simulink model "HSat_orbit"  (R2023a)
settings: Solver=FixedStepAuto  StartTime=0  StopTime=86400*900  MaxStep=3600  RelTol=1e-3  EnableMultiTasking=on
values from neighbouring files (symbols this model uses):
  ext_ENV_G = 6.674e-11    [HSat_op_setup.m]    (also in HSat_op_setup_merged_maria.m)
  ext_ENV_muEarth = 3.986005e14    (= 398600500000000)    [GEO_insertion_setup.m]    (also in HSat_op_setup.m; HSat_op_setup_merged_maria.m; init_orbit_analysis_with_drag_loss.m)
  ext_ENV_Re = 6.37813700*10^6    (= 6378137)    [HSat_op_setup.m]    (also in HSat_op_setup_merged_maria.m)
  ext_EOR_atmosphere_end = 1000e3    (= 1000000)    [HSat_op_setup.m]    (also in HSat_op_setup_merged_maria.m)
  ext_EOR_perigeeraise_end = 600e3    (= 600000)    [HSat_op_setup.m]    (also in HSat_op_setup_merged_maria.m)
  ext_Main_initDate_IC_T = sim_start    [HSat_op_setup.m]    (also in HSat_op_setup_merged_maria.m)
  ext_SC_activecorr_COE_ECI = [1, 1, 1, 0, 0, 0, 0, 0 ]    [HSat_op_setup.m]    (also in HSat_op_setup_merged_maria.m)
  ext_SC_balanced_COE_ECI = [ .500    0.70    1.100 1 1]    [HSat_op_setup.m]    (also in HSat_op_setup_merged_maria.m = [ 0.10 2.10 1.40    1.0000    1.0000]; launch_settings.m)
  ext_SC_cutofferror_COE_ECI = [150e3, .01, 0.1*pi/180, .1*pi/180,.1*pi/180, 0, 0, 0]    [HSat_op_setup.m]    (also in HSat_op_setup_merged_maria.m)
  ext_SC_init_COE_ECI = [a0,ecc0,i0,an0,ap0,tran0,eccan0,ma0]    [HSat_op_setup.m]    (also in HSat_op_setup_merged_maria.m)
  ext_SC_target_COE_ECI = [a1,ecc1,i1,an1,ap1,tran1,eccan1,ma1]    [HSat_op_setup.m]    (also in HSat_op_setup_merged_maria.m)
  ext_SC_target_lambda = 67*pi/180    (= 1.16937059884)    [HSat_op_setup.m]    (also in HSat_op_setup_merged_maria.m)
  sim_SC_init_CoG_EOR_dry = [-0.00448 0.00106 0.46931]    [HSat_op_setup.m]    (also in HSat_op_setup_merged_maria.m)
  sim_SC_init_CoG_propellant = [0 0 0.24758]    [HSat_op_setup.m]    (also in HSat_op_setup_merged_maria.m)
  sim_SC_init_dry_mass = sim_SC_init_wet_mass-sim_SC_init_propellant_mass    (= 727)    [HSat_op_setup.m]    (also in HSat_op_setup_merged_maria.m = 813.7)
  sim_SC_init_wet_mass = 750    [HSat_op_setup.m]    (also in HSat_op_setup_merged_maria.m)
  sim_thrust_force = [ ... (first row only)    [HSat_op_setup.m]    (also in HSat_op_setup_merged_maria.m)
  sim_thrust_massflow = [ ... (first row only)    [HSat_op_setup.m]    (also in HSat_op_setup_merged_maria.m)
  sim_thrust_vector = [ ... (first row only)    [HSat_op_setup.m]    (also in HSat_op_setup_merged_maria.m)
  sim_thruster_position = [ ... (first row only)    [HSat_op_setup.m]    (also in HSat_op_setup_merged_maria.m)
  sim_ts_save = 60    [HSat_op_setup.m]    (also in HSat_op_setup_merged_maria.m)
  third_body_jupiter = 1    [HSat_op_setup.m]    (also in HSat_op_setup_merged_maria.m)
  third_body_moon = 1    [HSat_op_setup.m]    (also in HSat_op_setup_merged_maria.m)
  third_body_sun = 1    [HSat_op_setup.m]    (also in HSat_op_setup_merged_maria.m)
libraries: aerolibutil x26, simulink x12, sharedtransform x7, sharedutil x4, Toolbox x3, matrix_library x1, simulink_extras x1
(part 2 of 5)

== system HSat_orbit/Subsystem1/Guidance/Subsystem1/Subsystem ==
  coe : Inport
  activecorr : Inport  Port=2
  coe1 : Inport  Port=3
  symelems : Inport  Port=4
  lambda1 : Inport  Port=5
  Abs : Abs  SaturateOnIntegerOverflow=off
  Bus Selector1 : BusSelector  OutputSignals=lambdadot,lambdaM
  Bus Selector2 : BusSelector  OutputSignals=sms
  Compare To Constant : simulink/Logic and Bit Operations/Compare To Constant  relop=<=  const=4  OutDataTypeStr=boolean
  Gain : Gain  Gain=180/pi
  Gain1 : Gain  Gain=180/pi
  Gain2 : Gain  Gain=180/pi
  Gain3 : Gain  Gain=.5
  Mux : Mux  Inputs=2
  Scope1 : Scope  NumInputPorts=3
  Scope2 : Scope  NumInputPorts=2
  Selector : Selector  InputPortWidth=8  IndexOptions=Index vector (dialog)  Indices=[2 3 4 5 6 7 8]  OutputSizes=1
  Subsystem1 : Subsystem
  Sum : Sum  Inputs=-+|
  plusminuspi : Subsystem
  NEARGEO : Outport
  ACTIVECORR : Outport  Port=2
  COE1 : Outport  Port=3
  wires:
  coe1/1 -> Selector/1
  coe/1 -> Bus Selector2/1
  lambda1/1 -> Sum/2
  symelems/1 -> Bus Selector1/1
  Abs/1 -> Compare To Constant/1
  Gain3/1 -> Gain1/1, Subsystem1/1(lambdadot_guide)
  Sum/1 -> plusminuspi/1(lambda)
  Selector/1 -> Mux/2
  Gain1/1 -> Scope1/2
  Gain2/1 -> Scope1/1
  Bus Selector1/1 -> Gain/1  "<lambdadot>"
  Bus Selector1/2 -> Sum/1  "<lambdaM>"
  Subsystem1/1(a_guide) -> Scope2/1, Mux/1
  Bus Selector2/1 -> Scope2/2  "<sms>"
  plusminuspi/1(lambdadot_guide) -> Gain2/1, Gain3/1
  Mux/1 -> COE1/1
  Gain/1 -> Scope1/3, Abs/1
  Compare To Constant/1 -> NEARGEO/1
  activecorr/1 -> ACTIVECORR/1

== system HSat_orbit/Subsystem1/Guidance/Subsystem1/perigeerraise ==
  coe : Inport
  "activecorr_coe " : Inport  Port=2
  Coe1 : Inport  Port=3
  Bus Selector : BusSelector  OutputSignals=sms
  Compare To Constant : simulink/Logic and Bit Operations/Compare To Constant  relop=<=  const=ext_EOR_perigeeraise_end  OutDataTypeStr=boolean
  Gain4 : Gain  Gain=[1 0 0 0 0 0 0 0]
  Gain5 : Gain  Gain=1.1
  Mux1 : Mux  Inputs=2
  Selector2 : Selector  InputPortWidth=8  IndexOptions=Index vector (dialog)  Indices=[2 3 4 5 6 7 8]  OutputSizes=1
  Subsystem2 : Subsystem
  Terminator : Terminator
  PERIGEEISLOW : Outport
  ACTIVECORR : Outport  Port=2
  COE1 : Outport  Port=3
  wires:
  Coe1/1 -> Selector2/1
  Compare To Constant/1 -> PERIGEEISLOW/1
  Subsystem2/2(Apogee altitude) -> Terminator/1
  "activecorr_coe "/1 -> Gain4/1
  Selector2/1 -> Mux1/2
  Subsystem2/1(Perigee altitude) -> Compare To Constant/1
  coe/1 -> Bus Selector/1, Subsystem2/1(COE)
  Gain4/1 -> ACTIVECORR/1
  Mux1/1 -> COE1/1
  Bus Selector/1 -> Gain5/1  "<sms>"
  Gain5/1 -> Mux1/1

== system HSat_orbit/Subsystem1/Navigation/Subsystem/Subsystem ==
  posECI : Inport
  velECI : Inport  Port=2
  Bus Creator : BusCreator  Inputs=11
  Demux : Demux  Outputs=11
  MATLAB Function : MATLAB Function  TreatAsAtomicUnit=on
  coe : Outport
  wires:
  posECI/1 -> MATLAB Function/1(r)
  Demux/10 -> Bus Creator/10  "truelong"
  Demux/1 -> Bus Creator/1  "sms"
  Demux/3 -> Bus Creator/3  "incl"
  Demux/7 -> Bus Creator/7  "eccan"
  Demux/9 -> Bus Creator/9  "arglat"
  Demux/4 -> Bus Creator/4  "raan"
  Demux/2 -> Bus Creator/2  "ecc"
  Demux/11 -> Bus Creator/11  "longper"
  Demux/6 -> Bus Creator/6  "truean"
  MATLAB Function/1(coe) -> Demux/1
  Bus Creator/1 -> coe/1  "coe"
  velECI/1 -> MATLAB Function/2(v)
  Demux/5 -> Bus Creator/5  "argp"
  Demux/8 -> Bus Creator/8  "meanan"

== system HSat_orbit/Subsystem1/Navigation/Subsystem/Subsystem2 ==
  jd : Inport
  epoch_jd : Inport  Port=2
  pos_ECI : Inport  Port=3
  vel_ECI : Inport  Port=4
  Bus Creator : BusCreator  Inputs=12
  Bus Creator1 : BusCreator  Inputs=10
  Bus Selector : BusSelector  OutputSignals=jd,epoch_jd,Raan,argp,nu,a,M,e,h
  Subsystem1 : Subsystem
  Subsystem7 : Subsystem
  Terminator : Terminator
  SyncElems : Outport
  wires:
  pos_ECI/1 -> Subsystem7/1(r)  "r"
  vel_ECI/1 -> Subsystem7/2(v)  "v"
  Subsystem7/9(e) -> Bus Creator/9
  Subsystem7/2(eabs) -> Bus Creator/2
  Subsystem7/10(h) -> Bus Creator/10
  Subsystem7/3(i) -> Bus Creator/3
  Subsystem7/5(argp) -> Bus Creator/5
  Subsystem7/4(Raan) -> Bus Creator/4
  Subsystem7/1(a) -> Bus Creator/1
  Subsystem7/6(nu) -> Bus Creator/6
  jd/1 -> Bus Creator/11  "jd"
  Bus Creator/1 -> Bus Selector/1
  Bus Selector/4 -> Subsystem1/4(<argp>)  "<argp>"
  Bus Selector/1 -> Subsystem1/1(<jd>)  "<jd>"
  Bus Selector/5 -> Subsystem1/5(<nu>)  "<nu>"
  Bus Selector/3 -> Subsystem1/3(<Raan>)  "<Raan>"
  Subsystem7/8(M) -> Bus Creator/8
  Subsystem7/7(E) -> Bus Creator/7
  Subsystem7/11(nu igen) -> Terminator/1
  epoch_jd/1 -> Bus Creator/12  "epoch_jd"
  Bus Selector/2 -> Subsystem1/2(epoch_jd)  "<epoch_jd>"
  Bus Selector/7 -> Subsystem1/7(M)  "<M>"
  Bus Selector/6 -> Subsystem1/6(a)  "<a>"
  Bus Selector/8 -> Subsystem1/8(e)  "<e>"
  Bus Selector/9 -> Subsystem1/9(h)  "<h>"
  Subsystem1/1(jd) -> Bus Creator1/1  "jd"
  Subsystem1/2(epochJd) -> Bus Creator1/2  "epochjd"
  Subsystem1/3(lambda) -> Bus Creator1/3  "lambda"
  Subsystem1/4(lambdaM) -> Bus Creator1/4  "lambdaM"
  Subsystem1/5(lambda0) -> Bus Creator1/5  "lambda0"
  Subsystem1/6(lambda_dot) -> Bus Creator1/6  "lambdadot"
  Subsystem1/7(ex) -> Bus Creator1/7  "ex"
  Subsystem1/9(ix) -> Bus Creator1/9  "ix"
  Bus Creator1/1 -> SyncElems/1
  Subsystem1/8(ey) -> Bus Creator1/8  "ey"
  Subsystem1/10(iy) -> Bus Creator1/10  "iy"

== system HSat_orbit/Subsystem1/Navigation/Subsystem8/Simplified Shadow Fraction ==
  note: Compute angular radius rho of Earth as viewed from ISS
  note: If dot product of normalized satellite position vector and sun vectors is smaller than cos rho then Earth is not blocking sun.
  x_sun_icrf : Inport  SampleTime=0
  X_icrf : Inport  Port=2
  Acos : Trigonometry  Operator=asin
  Acos1 : Trigonometry  Operator=cos
  Constant : Constant  Value=eps
  Constant1 : Constant  Value=eps
  Divide : Product  Inputs=/*
  Divide1 : Product  Inputs=*/
  Divide2 : Product  Inputs=/*
  Dot Product1 : DotProduct  OutDataTypeStr=Inherit: Inherit via internal rule
  Dot Product2 : DotProduct  OutDataTypeStr=Inherit: Inherit via internal rule
  Dot Product3 : DotProduct  OutDataTypeStr=Inherit: Inherit via internal rule
  Earth Radius : Constant  Value=ext_ENV_Re  VectorParams1D=off  SampleTime=0
  Gain : Gain  Gain=-1
  In Sun View : RelationalOperator  Operator=>  OutDataTypeStr=boolean  ZeroCross=off  RndMeth=Simplest  InputSameDT=off
  Max : MinMax  Function=max  Inputs=2
  Max1 : MinMax  Function=max  Inputs=2
  Sqrt1 : Sqrt
  Sqrt2 : Sqrt
  inView : Outport  SampleTime=0
  wires:
  Gain/1 -> Dot Product1/2, Divide/2, Dot Product1/1
  X_icrf/1 -> Divide2/2, Dot Product2/2, Dot Product2/1
  Earth Radius/1 -> Divide1/1
  Dot Product2/1 -> Sqrt1/1
  x_sun_icrf/1 -> Gain/1
  Max/1 -> Divide1/2, Divide2/1
  Divide1/1 -> Acos/1
  Acos/1 -> Acos1/1  "rho"
  Divide/1 -> Dot Product3/2
  Acos1/1 -> In Sun View/1
  Divide2/1 -> Dot Product3/1
  Dot Product3/1 -> In Sun View/2
  Dot Product1/1 -> Sqrt2/1
  Constant/1 -> Max/2
  In Sun View/1 -> inView/1
  Sqrt1/1 -> Max/1
  Sqrt2/1 -> Max1/1
  Max1/1 -> Divide/1
  Constant1/1 -> Max1/2

== system HSat_orbit/Subsystem1/Navigation/q_slo/VecNormalize ==
  In1 : Inport
  Constant : Constant
  Demux : Demux  Outputs=[-1 1]
  Divide : Product  Inputs=*/  OutDataTypeStr=double
  Ground : Ground
  Math Function : Math  Operator=square  SignedPower=on
  Math Function1 : Math  Operator=sqrt  SignedPower=on
  Mux : Mux  Inputs=2
  Mux1 : Mux  Inputs=2
  Product : Product  RndMeth=Zero
  Sum of Elements : Sum  Inputs=+
  Switch : Switch  Criteria=u2 > Threshold  Threshold=eps  SaturateOnIntegerOverflow=off  InputSameDT=off
  Out1 : Outport  VectorParamsAs1DForOutWhenUnconnected=off
  wires:
  Math Function/1 -> Sum of Elements/1
  Demux/1 -> Divide/1
  Constant/1 -> Mux1/2
  Mux1/1 -> Switch/3
  Divide/1 -> Out1/1
  Switch/1 -> Demux/1
  Mux/1 -> Switch/1
  Demux/2 -> Divide/2
  Product/1 -> Mux1/1
  In1/1 -> Product/1, Math Function/1, Mux/1
  Ground/1 -> Product/2
  Sum of Elements/1 -> Math Function1/1
  Math Function1/1 -> Mux/2, Switch/2

== system HSat_orbit/Subsystem1/Navigation/q_slo/VecNormalize1 ==
  In1 : Inport
  Constant : Constant
  Demux : Demux  Outputs=[-1 1]
  Divide : Product  Inputs=*/  OutDataTypeStr=double
  Ground : Ground
  Math Function : Math  Operator=square  SignedPower=on
  Math Function1 : Math  Operator=sqrt  SignedPower=on
  Mux : Mux  Inputs=2
  Mux1 : Mux  Inputs=2
  Product : Product  RndMeth=Zero
  Sum of Elements : Sum  Inputs=+
  Switch : Switch  Criteria=u2 > Threshold  Threshold=eps  SaturateOnIntegerOverflow=off  InputSameDT=off
  Out1 : Outport  VectorParamsAs1DForOutWhenUnconnected=off
  wires:
  Math Function/1 -> Sum of Elements/1
  Demux/1 -> Divide/1
  Constant/1 -> Mux1/2
  Mux1/1 -> Switch/3
  Divide/1 -> Out1/1
  Switch/1 -> Demux/1
  Mux/1 -> Switch/1
  Demux/2 -> Divide/2
  Product/1 -> Mux1/1
  In1/1 -> Product/1, Math Function/1, Mux/1
  Ground/1 -> Product/2
  Sum of Elements/1 -> Math Function1/1
  Math Function1/1 -> Mux/2, Switch/2

== system HSat_orbit/Subsystem1/Navigation/q_slo/VecNormalize2 ==
  In1 : Inport
  Constant : Constant
  Demux : Demux  Outputs=[-1 1]
  Divide : Product  Inputs=*/  OutDataTypeStr=double
  Ground : Ground
  Math Function : Math  Operator=square  SignedPower=on
  Math Function1 : Math  Operator=sqrt  SignedPower=on
  Mux : Mux  Inputs=2
  Mux1 : Mux  Inputs=2
  Product : Product  RndMeth=Zero
  Sum of Elements : Sum  Inputs=+
  Switch : Switch  Criteria=u2 > Threshold  Threshold=eps  SaturateOnIntegerOverflow=off  InputSameDT=off
  Out1 : Outport  VectorParamsAs1DForOutWhenUnconnected=off
  wires:
  Math Function/1 -> Sum of Elements/1
  Demux/1 -> Divide/1
  Constant/1 -> Mux1/2
  Mux1/1 -> Switch/3
  Divide/1 -> Out1/1
  Switch/1 -> Demux/1
  Mux/1 -> Switch/1
  Demux/2 -> Divide/2
  Product/1 -> Mux1/1
  In1/1 -> Product/1, Math Function/1, Mux/1
  Ground/1 -> Product/2
  Sum of Elements/1 -> Math Function1/1
  Math Function1/1 -> Mux/2, Switch/2

== system HSat_orbit/Subsystem1/Navigation/q_slo/VecNormalize3 ==
  In1 : Inport
  Constant : Constant
  Demux : Demux  Outputs=[-1 1]
  Divide : Product  Inputs=*/  OutDataTypeStr=double
  Ground : Ground
  Math Function : Math  Operator=square  SignedPower=on
  Math Function1 : Math  Operator=sqrt  SignedPower=on
  Mux : Mux  Inputs=2
  Mux1 : Mux  Inputs=2
  Product : Product  RndMeth=Zero
  Sum of Elements : Sum  Inputs=+
  Switch : Switch  Criteria=u2 > Threshold  Threshold=eps  SaturateOnIntegerOverflow=off  InputSameDT=off
  Out1 : Outport  VectorParamsAs1DForOutWhenUnconnected=off
  wires:
  Math Function/1 -> Sum of Elements/1
  Demux/1 -> Divide/1
  Constant/1 -> Mux1/2
  Mux1/1 -> Switch/3
  Divide/1 -> Out1/1
  Switch/1 -> Demux/1
  Mux/1 -> Switch/1
  Demux/2 -> Divide/2
  Product/1 -> Mux1/1
  In1/1 -> Product/1, Math Function/1, Mux/1
  Ground/1 -> Product/2
  Sum of Elements/1 -> Math Function1/1
  Math Function1/1 -> Mux/2, Switch/2

== system HSat_orbit/Subsystem1/Navigation/q_slo/Z x R ==
  a(1) a(2) a(3) : Inport
  b(1) b(2) b(3) : Inport  Port=2
  Product : Product  InputSameDT=on  SaturateOnIntegerOverflow=on  OutDataTypeStr=Inherit: Same as first input
  Product1 : Product  InputSameDT=on  SaturateOnIntegerOverflow=on  OutDataTypeStr=Inherit: Same as first input
  Selector : Selector  InputPortWidth=3  IndexOptions=Index vector (dialog)  Indices=[2 3 1]  OutputSizes=1
  Selector1 : Selector  InputPortWidth=3  IndexOptions=Index vector (dialog)  Indices=[3 1 2]  OutputSizes=1
  Selector2 : Selector  InputPortWidth=3  IndexOptions=Index vector (dialog)  Indices=[2 3 1]  OutputSizes=1
  Selector3 : Selector  InputPortWidth=3  IndexOptions=Index vector (dialog)  Indices=[3 1 2]  OutputSizes=1
  Sum : Sum  Inputs=+|-  InputSameDT=on  SaturateOnIntegerOverflow=on  OutDataTypeStr=Inherit: Same as first input
  c(1) c(2) c(3) : Outport  InitialOutput=0
  wires:
  Selector3/1 -> Product1/1
  Selector2/1 -> Product1/2
  Product1/1 -> Sum/2
  Selector1/1 -> Product/2
  Product/1 -> Sum/1
  a(1) a(2) a(3)/1 -> Selector3/1, Selector/1
  Selector/1 -> Product/1
  b(1) b(2) b(3)/1 -> Selector2/1, Selector1/1
  Sum/1 -> c(1) c(2) c(3)/1

== system HSat_orbit/Subsystem1/Navigation/q_slo/Z x Y ==
  a(1) a(2) a(3) : Inport
  b(1) b(2) b(3) : Inport  Port=2
  Product : Product  InputSameDT=on  SaturateOnIntegerOverflow=on  OutDataTypeStr=Inherit: Same as first input
  Product1 : Product  InputSameDT=on  SaturateOnIntegerOverflow=on  OutDataTypeStr=Inherit: Same as first input
  Selector : Selector  InputPortWidth=3  IndexOptions=Index vector (dialog)  Indices=[2 3 1]  OutputSizes=1
  Selector1 : Selector  InputPortWidth=3  IndexOptions=Index vector (dialog)  Indices=[3 1 2]  OutputSizes=1
  Selector2 : Selector  InputPortWidth=3  IndexOptions=Index vector (dialog)  Indices=[2 3 1]  OutputSizes=1
  Selector3 : Selector  InputPortWidth=3  IndexOptions=Index vector (dialog)  Indices=[3 1 2]  OutputSizes=1
  Sum : Sum  Inputs=+|-  InputSameDT=on  SaturateOnIntegerOverflow=on  OutDataTypeStr=Inherit: Same as first input
  c(1) c(2) c(3) : Outport  InitialOutput=0
  wires:
  Selector3/1 -> Product1/1
  Selector2/1 -> Product1/2
  Product1/1 -> Sum/2
  Selector1/1 -> Product/2
  Product/1 -> Sum/1
  a(1) a(2) a(3)/1 -> Selector3/1, Selector/1
  Selector/1 -> Product/1
  b(1) b(2) b(3)/1 -> Selector2/1, Selector1/1
  Sum/1 -> c(1) c(2) c(3)/1

== system HSat_orbit/Subsystem1/Subsystem4/EORattitude/Subsystem ==
  AmomECI : Inport
  q_eci2scb : Inport  Port=2
  EORthrustSCB : Inport  Port=3
  EORtorqueSCB : Inport  Port=4
  thrust_slo : Inport  Port=5
  q_slo2eci : Inport  Port=6
  sunv_eci : Inport  Port=7
  Quaternion Rotation1 : aerolibutil/Quaternion Rotation
  Subsystem1 : Subsystem
  Subsystem3 : Subsystem
  qECI2scb : Outport
  DoAMOM : Outport  Port=2
  NoAMOM : Outport  Port=3
  wires:
  q_slo2eci/1 -> Subsystem1/4(q_slo2eci)
  EORthrustSCB/1 -> Subsystem1/2(EORthrustSCB)
  sunv_eci/1 -> Subsystem1/5(sunv_eci)
  EORtorqueSCB/1 -> Subsystem3/2(EORtorqueSCB)
  thrust_slo/1 -> Subsystem1/3(thrust_slo)
  AmomECI/1 -> Quaternion Rotation1/2
  Subsystem1/1(qECI2scb) -> qECI2scb/1
  Subsystem3/3(FlipPlusMinus) -> Subsystem1/1(Flipsign)
  Quaternion Rotation1/1 -> Subsystem3/1(AmomSCB)  "amomscb"
  q_eci2scb/1 -> Quaternion Rotation1/1
  Subsystem3/1(DoAMOM) -> DoAMOM/1
  Subsystem3/2(NoAMOM) -> NoAMOM/1

== system HSat_orbit/Subsystem1/Subsystem4/EORattitude/Subsystem2 ==
  PPU1active : Inport
  AllThrustsSCB : Inport  Port=2
  PPU2active : Inport  Port=3
  AllTorquesSCB1 : Inport  Port=4
  PPU1ORTHR : Inport  Port=5
  PPU2ORTHR : Inport  Port=6
  Logical Operator : Logic  AllPortsSameDT=off  OutDataTypeStr=boolean
  Logical Operator1 : Logic  AllPortsSameDT=off  OutDataTypeStr=boolean
  Logical Operator2 : Logic  Operator=OR  AllPortsSameDT=off  OutDataTypeStr=boolean
  PPU1 : Subsystem
  PPU3 : Subsystem
  Product{,1..3} (4 alike) : Product
  Subsystem1 : Subsystem
  Sum1 : Sum  Inputs=++|
  Sum2 : Sum  Inputs=++|
  ActiveThrusters : Outport
  EORForceSCB : Outport  Port=2
  EORTorqueSCB : Outport  Port=3
  wires:
  AllTorquesSCB1/1 -> Subsystem1/2(AllTorquesSCB)
  Sum1/1 -> EORForceSCB/1
  Product2/1 -> Sum2/1
  PPU3/2(TorqueSCB) -> Product3/2
  PPU3/1(ForceSCB) -> Product1/2
  Sum2/1 -> EORTorqueSCB/1
  PPU1/1(ForceSCB) -> Product/2
  Subsystem1/2(TorquesORSCB) -> PPU3/3(TorqueORSCB), PPU1/3(TorqueORSCB)
  PPU1/2(TorqueSCB) -> Product2/2
  PPU2ORTHR/1 -> PPU3/2(OR ThrustNo)
  Logical Operator2/1 -> ActiveThrusters/1
  Subsystem1/1(ForceORSCB) -> PPU3/1(ForceORSCB), PPU1/1(ForceORSCB)
  PPU3/3(activethrusters) -> Logical Operator1/2
  AllThrustsSCB/1 -> Subsystem1/1(AllForcesSCB)
  Logical Operator/1 -> Logical Operator2/1
  PPU2active/1 -> Product3/1, Logical Operator1/1, Product1/1
  Product1/1 -> Sum1/2
  Logical Operator1/1 -> Logical Operator2/2
  Product/1 -> Sum1/1
  PPU1/3(activethrusters) -> Logical Operator/2
  PPU1active/1 -> Product2/1, Logical Operator/1, Product/1
  PPU1ORTHR/1 -> PPU1/2(OR ThrustNo)
  Product3/1 -> Sum2/2

== system HSat_orbit/Subsystem1/Subsystem4/EORattitude/Subsystem4 ==
  AmomECI : Inport
  EORthrustSCB : Inport  Port=2
  EORtorqueSCB : Inport  Port=3
  thrust_slo : Inport  Port=4
  q_slo2eci : Inport  Port=5
  sunv_eci : Inport  Port=6
  Delay1 : Delay  DelayLength=1  InitialConditionSource=Input port  InitialCondition=0
      settings: InputPortMap=u0,p4
  Quaternion Multiplication2 : aerolibutil/Quaternion Multiplication
  Quaternion Rotation1 : aerolibutil/Quaternion Rotation
  Subsystem1 : Subsystem
  Subsystem2 : Subsystem
  Subsystem3 : Subsystem
  Subsystem4 : Subsystem
  Switch1 : Switch  Criteria=u2 > Threshold  SaturateOnIntegerOverflow=off  InputSameDT=off
  qECI2scb : Outport
  DoAMOM : Outport  Port=2
  NoAMOM : Outport  Port=3
  wires:
  AmomECI/1 -> Quaternion Rotation1/2
  Quaternion Rotation1/1 -> Subsystem3/1(AmomSCB)  "amomscb"
  EORthrustSCB/1 -> Subsystem1/4(thrustscb), Subsystem2/1(thrustscb)  "thrustscb"
  EORtorqueSCB/1 -> Subsystem3/2(EORtorqueSCB)
  Subsystem3/1(Flipyaxis) -> Switch1/2
  Subsystem2/1(qflipscb) -> Switch1/1
  Subsystem4/1(qflipscb) -> Switch1/3
  Switch1/1 -> Quaternion Multiplication2/2
  Quaternion Multiplication2/1 -> Delay1/1, qECI2scb/1
  Delay1/1 -> Quaternion Rotation1/1
  Subsystem1/1(q*r) -> Delay1/2, Quaternion Multiplication2/1
  q_slo2eci/1 -> Subsystem1/1(q)
  thrust_slo/1 -> Subsystem1/2(vec)
  sunv_eci/1 -> Subsystem1/3(sunvECI)
  Subsystem3/2(DoAMOM) -> DoAMOM/1
  Subsystem3/3(NoAMOM) -> NoAMOM/1

== system HSat_orbit/Subsystem1/Subsystem4/Subsystem6/Subsystem2 ==
  PPU1active : Inport
  PPU2active : Inport  Port=2
  AllTorquesSCB : Inport  Port=3
  q_eci2scb_wanted : Inport  Port=4
  WantedTorqueECI : Inport  Port=5
  sunv : Inport  Port=6
  Multiport Switch : MultiPortSwitch  SaturateOnIntegerOverflow=off  InputSameDT=off
  Multiport Switch1 : MultiPortSwitch  SaturateOnIntegerOverflow=off  InputSameDT=off
  PPU1 : Subsystem
  PPU1+2 : Subsystem
  PPU2 : Subsystem
  Subsystem : Subsystem
  Subsystem1 : Subsystem
  Sum1 : Sum  Inputs=++|
  ActiveThrusters : Outport
  q_eci2scb : Outport  Port=2
  wires:
  Multiport Switch1/1 -> ActiveThrusters/1
  PPU1active/1 -> Sum1/1
  PPU2active/1 -> Sum1/2
  PPU1+2/2(activethrusters) -> Multiport Switch1/4
  PPU1/2(activethrusters) -> Multiport Switch1/2
  PPU1/1(torqueSCB) -> Multiport Switch/2  "torquescb"
  PPU1+2/1(torqueSCB) -> Multiport Switch/4  "torquescb"
  PPU2/2(activethrusters) -> Multiport Switch1/3
  Sum1/1 -> Multiport Switch/1, Multiport Switch1/1
  WantedTorqueECI/1 -> Subsystem1/2(WantedTorqueECI), PPU1+2/2(WantedTorqueECI), PPU2/2(WantedTorqueECI), PPU1/2(WantedTorqueECI)
  PPU2/1(torqueSCB) -> Multiport Switch/3  "torquescb"
  Subsystem/1(TorqueSKECI) -> PPU1+2/1(TorqueSKECI), PPU2/1(TorqueSKECI), PPU1/1(TorqueSKECI)
  q_eci2scb_wanted/1 -> Subsystem/2(q_eci2scb_wanted)
  AllTorquesSCB/1 -> Subsystem/1(AllTorquesSCB)
  Subsystem1/1(q_eci2scb) -> q_eci2scb/1
  sunv/1 -> Subsystem1/3(sunvECI)
  Multiport Switch/1 -> Subsystem1/1(TorqueSCB)

== system HSat_orbit/Subsystem1/Subsystem4/TorquesAndForces/Subsystem ==
  SC_mass : Inport
  Constant1 : Constant  Value=sim_SC_init_CoG_EOR_dry
  Constant2 : Constant  Value=sim_SC_init_CoG_propellant
  Constant3 : Constant  Value=sim_SC_init_wet_mass
  Constant4 : Constant  Value=sim_SC_init_dry_mass
  Divide : Product  Inputs=/*
  Product : Product
  Product1 : Product
  Reshape : Reshape  OutputDimensionality=Row vector (2-D)
  Sum : Sum  Inputs=+-|
  Sum1 : Sum  Inputs=+|+
  SC_CoG : Outport
  wires:
  Constant4/1 -> Sum/2
  Product1/1 -> Sum1/2
  Constant3/1 -> Product1/1
  SC_mass/1 -> Divide/1, Sum/1
  Constant1/1 -> Product1/2
  Product/1 -> Sum1/1
  Sum1/1 -> Divide/2
  Constant2/1 -> Product/2
  Sum/1 -> Product/1
  Divide/1 -> Reshape/1
  Reshape/1 -> SC_CoG/1

== system HSat_orbit/Subsystem1/Dynamics/Subsystem/3 body perturbation legendre polynomial/Subsystem1 ==
  sat : Inport
  3 body : Inport  Port=2
  mass : Inport  Port=3
  Legendre deg : Inport  Port=4
  Constant : Constant  Value=6.6743e-11
  Divide : Product  Inputs=/*
  Divide1 : Product  Inputs=*/
  Dot Product : DotProduct  OutDataTypeStr=Inherit: Inherit via internal rule
  Dot Product1 : DotProduct  OutDataTypeStr=Inherit: Inherit via internal rule
  Dot Product2 : DotProduct  OutDataTypeStr=Inherit: Inherit via internal rule
  MATLAB Function : MATLAB Function  TreatAsAtomicUnit=on
  Product{,1..3} (4 alike) : Product
  Sqrt : Sqrt
  Sqrt1 : Sqrt
  Subtract : Sum  Inputs=-+
  Subtract1 : Sum  Inputs=+-
  cos angle : Subsystem
  Out1 : Outport
  wires:
  sat/1 -> cos angle/1(sat), Subtract/2, Subtract1/2, Dot Product2/2, Dot Product2/1  "r_sat"
  3 body/1 -> Dot Product1/1, Dot Product/2, Dot Product/1, Dot Product1/2, Subtract1/1, cos angle/2(3 body)  "r_3body"
  cos angle/1(cos angle) -> MATLAB Function/1(costheta)
  Legendre deg/1 -> MATLAB Function/2(degree)
  Divide/1 -> MATLAB Function/3(h)
  mass/1 -> Product/2
  Constant/1 -> Product/1
  Product/1 -> Divide1/1  "mu_3body"
  Divide1/1 -> Product1/1
  Product1/1 -> Out1/1
  MATLAB Function/1(beta) -> Product2/1
  Subtract1/1 -> Product2/2  "r_sat3body"
  Product2/1 -> Subtract/1
  Subtract/1 -> Product1/2
  Dot Product/1 -> Product3/1
  Product3/1 -> Divide1/2
  Dot Product1/1 -> Sqrt/1
  Sqrt/1 -> Divide/1, Product3/2  "| r_3body |"
  Dot Product2/1 -> Sqrt1/1
  Sqrt1/1 -> Divide/2  "| r_sat |"

== system HSat_orbit/Subsystem1/Dynamics/Subsystem/3 body perturbation legendre polynomial/Subsystem2 ==
  sat : Inport
  3 body : Inport  Port=2
  mass : Inport  Port=3
  Legendre deg : Inport  Port=4
  Constant : Constant  Value=ext_ENV_G
  Divide : Product  Inputs=/*
  Divide1 : Product  Inputs=*/
  Dot Product : DotProduct  OutDataTypeStr=Inherit: Inherit via internal rule
  Dot Product1 : DotProduct  OutDataTypeStr=Inherit: Inherit via internal rule
  Dot Product2 : DotProduct  OutDataTypeStr=Inherit: Inherit via internal rule
  MATLAB Function : MATLAB Function  TreatAsAtomicUnit=on
  Product{,1..3} (4 alike) : Product
  Sqrt : Sqrt
  Sqrt1 : Sqrt
  Subtract : Sum  Inputs=-+
  Subtract1 : Sum  Inputs=+-
  cos angle : Subsystem
  Out1 : Outport
  wires:
  sat/1 -> cos angle/1(sat), Subtract/2, Subtract1/2, Dot Product2/2, Dot Product2/1  "r_sat"
  3 body/1 -> Dot Product1/1, Dot Product/2, Dot Product/1, Dot Product1/2, Subtract1/1, cos angle/2(3 body)  "r_3body"
  cos angle/1(cos angle) -> MATLAB Function/1(costheta)
  Legendre deg/1 -> MATLAB Function/2(degree)
  Divide/1 -> MATLAB Function/3(h)
  mass/1 -> Product/2
  Constant/1 -> Product/1
  Product/1 -> Divide1/1  "mu_3body"
  Divide1/1 -> Product1/1
  Product1/1 -> Out1/1
  MATLAB Function/1(beta) -> Product2/1
  Subtract1/1 -> Product2/2  "r_sat3body"
  Product2/1 -> Subtract/1
  Subtract/1 -> Product1/2
  Dot Product/1 -> Product3/1
  Product3/1 -> Divide1/2
  Dot Product1/1 -> Sqrt/1
  Sqrt/1 -> Divide/1, Product3/2  "| r_3body |"
  Dot Product2/1 -> Sqrt1/1
  Sqrt1/1 -> Divide/2  "| r_sat |"

== system HSat_orbit/Subsystem1/Dynamics/Subsystem/3 body perturbation legendre polynomial/Subsystem3 ==
  sat : Inport
  3 body : Inport  Port=2
  mass : Inport  Port=3
  Legendre deg : Inport  Port=4
  Constant : Constant  Value=6.6743e-11
  Divide : Product  Inputs=/*
  Divide1 : Product  Inputs=*/
  Dot Product : DotProduct  OutDataTypeStr=Inherit: Inherit via internal rule
  Dot Product1 : DotProduct  OutDataTypeStr=Inherit: Inherit via internal rule
  Dot Product2 : DotProduct  OutDataTypeStr=Inherit: Inherit via internal rule
  MATLAB Function : MATLAB Function  TreatAsAtomicUnit=on
  Product{,1..3} (4 alike) : Product
  Sqrt : Sqrt
  Sqrt1 : Sqrt
  Subtract : Sum  Inputs=-+
  Subtract1 : Sum  Inputs=+-
  cos angle : Subsystem
  Out1 : Outport
  wires:
  sat/1 -> cos angle/1(sat), Subtract/2, Subtract1/2, Dot Product2/2, Dot Product2/1  "r_sat"
  3 body/1 -> Dot Product1/1, Dot Product/2, Dot Product/1, Dot Product1/2, Subtract1/1, cos angle/2(3 body)  "r_3body"
  cos angle/1(cos angle) -> MATLAB Function/1(costheta)
  Legendre deg/1 -> MATLAB Function/2(degree)
  Divide/1 -> MATLAB Function/3(h)
  mass/1 -> Product/2
  Constant/1 -> Product/1
  Product/1 -> Divide1/1  "mu_3body"
  Divide1/1 -> Product1/1
  Product1/1 -> Out1/1
  MATLAB Function/1(beta) -> Product2/1
  Subtract1/1 -> Product2/2  "r_sat3body"
  Product2/1 -> Subtract/1
  Subtract/1 -> Product1/2
  Dot Product/1 -> Product3/1
  Product3/1 -> Divide1/2
  Dot Product1/1 -> Sqrt/1
  Sqrt/1 -> Divide/1, Product3/2  "| r_3body |"
  Dot Product2/1 -> Sqrt1/1
  Sqrt1/1 -> Divide/2  "| r_sat |"

== system HSat_orbit/Subsystem1/Guidance/Subsystem1/Subsystem/Subsystem1 ==
  lambdadot_guide : Inport
  Constant1 : Constant  Value=2*pi
  Constant5 : Constant  Value=2*pi*86164
  Constant6 : Constant  Value=ext_ENV_muEarth
  Constant7 : Constant  Value=1/3
  Constant8 : Constant  Value=2*pi
  Divide1 : Product  Inputs=**
  Divide2 : Product  Inputs=*/
  Divide3 : Product  Inputs=*/
  Gain : Gain
  Math Function4 : Math  Operator=square
  Math Function5 : Math  Operator=pow
  Subtract1 : Sum
  a_guide : Outport
  wires:
  Constant6/1 -> Divide1/2
  Divide1/1 -> Math Function5/1
  Constant7/1 -> Math Function5/2
  lambdadot_guide/1 -> Gain/1
  Math Function4/1 -> Divide1/1
  Math Function5/1 -> a_guide/1
  Constant8/1 -> Subtract1/2
  Subtract1/1 -> Divide2/2
  Divide2/1 -> Divide3/1  "T-period"
  Constant5/1 -> Divide2/1
  Constant1/1 -> Divide3/2
  Divide3/1 -> Math Function4/1  "T-period"
  Gain/1 -> Subtract1/1

== system HSat_orbit/Subsystem1/Guidance/Subsystem1/Subsystem/plusminuspi ==
  lambda : Inport
  Constant1 : Constant  Value=2*pi
  Constant2 : Constant  Value=2*pi
  Constant4 : Constant  Value=2*pi
  Constant5 : Constant  Value=pi
  Math Function1 : Math  Operator=mod
  Math Function2 : Math  Operator=mod
  Math Function3 : Math  Operator=mod
  Sum11 : Sum  Inputs=|+-
  Sum12 : Sum  Inputs=|++
  lambdadot_guide : Outport
  wires:
  Sum11/1 -> Math Function1/1
  Sum12/1 -> Math Function3/1
  Math Function3/1 -> Sum11/1
  Constant5/1 -> Sum12/2, Sum11/2
  Constant4/1 -> Math Function3/2
  lambda/1 -> Math Function2/1
  Constant1/1 -> Math Function1/2
  Math Function2/1 -> Sum12/1
  Constant2/1 -> Math Function2/2
  Math Function1/1 -> lambdadot_guide/1

== system HSat_orbit/Subsystem1/Guidance/Subsystem1/perigeerraise/Subsystem2 ==
  COE : Inport
  Bus Selector : BusSelector  OutputSignals=sms,ecc
  Constant : Constant
  Constant1 : Constant  Value=ext_ENV_Re
  Product : Product
  Product1 : Product
  Sum : Sum  Inputs=|-+
  Sum1 : Sum  Inputs=|++
  Sum2 : Sum  Inputs=|+-
  Sum3 : Sum  Inputs=|+-
  Perigee altitude : Outport
  Apogee altitude : Outport  Port=2
  wires:
  Product1/1 -> Sum3/1
  COE/1 -> Bus Selector/1
  Sum1/1 -> Product1/2
  Product/1 -> Sum2/1
  Constant/1 -> Sum1/2, Sum/2
  Sum/1 -> Product/2
  Bus Selector/1 -> Product1/1, Product/1  "<sms>"
  Sum2/1 -> Perigee altitude/1
  Sum3/1 -> Apogee altitude/1
  Constant1/1 -> Sum2/2, Sum3/2
  Bus Selector/2 -> Sum/1, Sum1/1  "<ecc>"

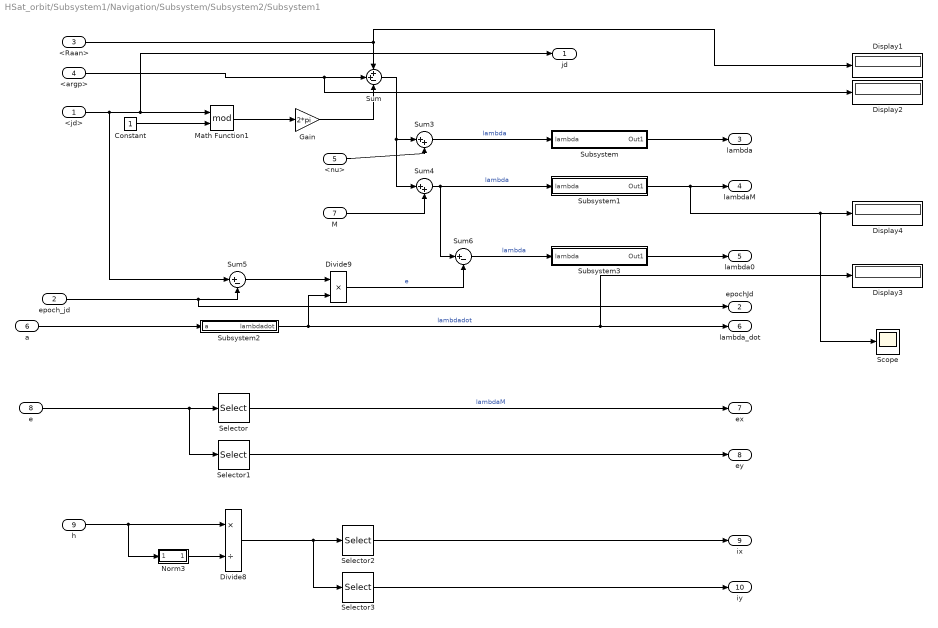
== system HSat_orbit/Subsystem1/Navigation/Subsystem/Subsystem2/Subsystem1 ==
  <jd> : Inport
  epoch_jd : Inport  Port=2
  <Raan> : Inport  Port=3
  <argp> : Inport  Port=4
  <nu> : Inport  Port=5
  a : Inport  Port=6
  M : Inport  Port=7
  e : Inport  Port=8
  h : Inport  Port=9
  Constant : Constant
  Display{1..4} (4 alike) : Display
  Divide8 : Product  Inputs=*/
  Divide9 : Product  Inputs=**
  Gain : Gain  Gain=2*pi
  Math Function1 : Math  Operator=mod
  Norm3 : Subsystem  Tag=||u||
      mask Display: disp('||u||')
  Scope : Scope
  Selector : Selector  InputPortWidth=3  IndexOptions=Index vector (dialog)  Indices=[1]  OutputSizes=1
  Selector1 : Selector  InputPortWidth=3  IndexOptions=Index vector (dialog)  Indices=[2]  OutputSizes=1
  Selector2 : Selector  InputPortWidth=3  IndexOptions=Index vector (dialog)  Indices=[1]  OutputSizes=1
  Selector3 : Selector  InputPortWidth=3  IndexOptions=Index vector (dialog)  Indices=[2]  OutputSizes=1
  Subsystem : Subsystem
  Subsystem1 : Subsystem
  Subsystem2 : Subsystem
  Subsystem3 : Subsystem
  Sum : Sum  Inputs=++-
  Sum3 : Sum  Inputs=|++
  Sum4 : Sum  Inputs=|++
  Sum5 : Sum  Inputs=|+-
  Sum6 : Sum  Inputs=|+-
  jd : Outport
  epochJd : Outport  Port=2
  lambda : Outport  Port=3
  lambdaM : Outport  Port=4
  lambda0 : Outport  Port=5
  lambda_dot : Outport  Port=6
  ex : Outport  Port=7
  ey : Outport  Port=8
  ix : Outport  Port=9
  iy : Outport  Port=10
  wires:
  <Raan>/1 -> Sum/1, Display1/1
  <nu>/1 -> Sum3/2
  Gain/1 -> Sum/3
  Math Function1/1 -> Gain/1
  <jd>/1 -> Sum5/1, Math Function1/1, jd/1
  Constant/1 -> Math Function1/2
  a/1 -> Subsystem2/1(a)
  Sum/1 -> Sum4/1, Sum3/1
  M/1 -> Sum4/2
  epoch_jd/1 -> epochJd/1, Sum5/2
  Sum5/1 -> Divide9/1
  Subsystem2/1(lambdadot) -> Divide9/2, Display3/1, lambda_dot/1  "lambdadot"
  Divide9/1 -> Sum6/2  "e"
  e/1 -> Selector1/1, Selector/1
  Selector1/1 -> ey/1
  Selector/1 -> ex/1  "lambdaM"
  Divide8/1 -> Selector3/1, Selector2/1
  Selector3/1 -> iy/1
  Selector2/1 -> ix/1
  Norm3/1(Out1) -> Divide8/2
  h/1 -> Norm3/1(In1), Divide8/1
  Sum4/1 -> Sum6/1, Subsystem1/1(lambda)  "lambda"
  Sum3/1 -> Subsystem/1(lambda)  "lambda"
  Subsystem/1(Out1) -> lambda/1
  Subsystem1/1(Out1) -> Scope/1, Display4/1, lambdaM/1
  Sum6/1 -> Subsystem3/1(lambda)  "lambda"
  Subsystem3/1(Out1) -> lambda0/1
  <argp>/1 -> Display2/1, Sum/2

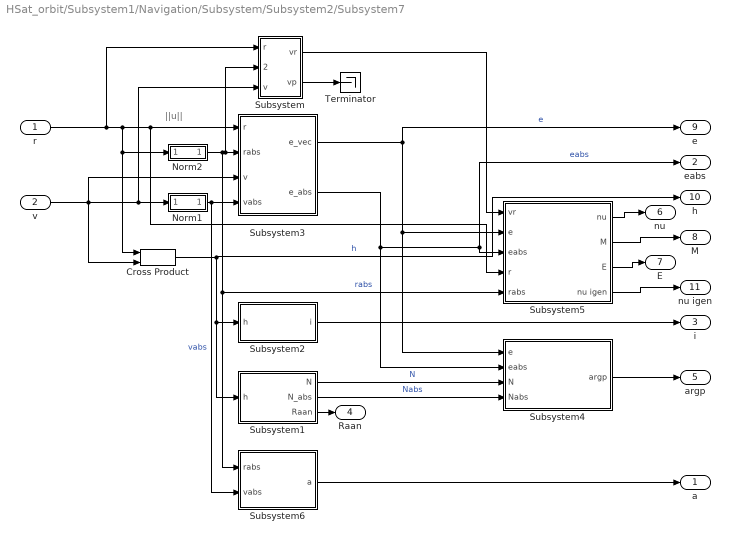
== system HSat_orbit/Subsystem1/Navigation/Subsystem/Subsystem2/Subsystem7 ==
  note: ||u||
  r : Inport
  v : Inport  Port=2
  Cross Product : matrix_library/Cross Product
  Norm1 : Subsystem  Tag=||u||
      mask Display: disp('||u||')
  Norm2 : Subsystem  Tag=||u||
      mask Display: disp('||u||')
  Subsystem : Subsystem
  Subsystem1 : Subsystem
  Subsystem2 : Subsystem
  Subsystem3 : Subsystem
  Subsystem4 : Subsystem
  Subsystem5 : Subsystem
  Subsystem6 : Subsystem
  Terminator : Terminator
  a : Outport
  eabs : Outport  Port=2
  i : Outport  Port=3
  Raan : Outport  Port=4
  argp : Outport  Port=5
  nu : Outport  Port=6
  E : Outport  Port=7
  M : Outport  Port=8
  e : Outport  Port=9
  h : Outport  Port=10
  nu igen : Outport  Port=11
  wires:
  Subsystem5/1(nu) -> nu/1
  Subsystem1/3(Raan) -> Raan/1
  Subsystem1/1(N) -> Subsystem4/3(N)  "N"
  Subsystem6/1(a) -> a/1
  Subsystem1/2(N_abs) -> Subsystem4/4(Nabs)  "Nabs"
  Subsystem3/1(e_vec) -> e/1, Subsystem4/1(e), Subsystem5/2(e)  "e"
  Subsystem4/1(argp) -> argp/1
  Norm1/1(Out1) -> Subsystem6/2(vabs), Subsystem3/4(vabs)  "vabs"
  Subsystem2/1(i) -> i/1
  Cross Product/1 -> Subsystem1/1(h), Subsystem2/1(h), h/1  "h"
  v/1 -> Cross Product/2, Subsystem3/3(v), Subsystem/3(v), Norm1/1(In1)
  Subsystem3/2(e_abs) -> eabs/1, Subsystem5/3(eabs), Subsystem4/2(eabs)  "eabs"
  Norm2/1(Out1) -> Subsystem/2(rabs), Subsystem3/2(rabs), Subsystem6/1(rabs), Subsystem5/5(rabs)  "rabs"
  Subsystem5/2(M) -> M/1
  Subsystem5/4(nu igen) -> nu igen/1
  Subsystem5/3(E) -> E/1
  r/1 -> Subsystem/1(r), Norm2/1(In1), Cross Product/1, Subsystem5/4(r), Subsystem3/1(r)
  Subsystem/1(vr) -> Subsystem5/1(vr)
  Subsystem/2(vp) -> Terminator/1

== system HSat_orbit/Subsystem1/Subsystem4/EORattitude/Subsystem/Subsystem1 ==
  note: the scbp fram is an intemediate frame where:
      | - z is aligned with the resutling thrust,
      | - y is the normalised cross product between the sun vector and z
      | - x completes the orthogonal system
  Flipsign : Inport
  EORthrustSCB : Inport  Port=2
  thrust_slo : Inport  Port=3
  q_slo2eci : Inport  Port=4
  sunv_eci : Inport  Port=5
  Quaternion Inverse : aerolibutil/Quaternion Inverse
  Quaternion Multiplication : aerolibutil/Quaternion Multiplication
  Quaternion Rotation : aerolibutil/Quaternion Rotation
  Subsystem : Subsystem
  q_scb_calc : Subsystem
  qECI2scb : Outport
  wires:
  thrust_slo/1 -> Quaternion Rotation/2
  q_slo2eci/1 -> Quaternion Inverse/1
  sunv_eci/1 -> q_scb_calc/2(sunvECI)
  Quaternion Rotation/1 -> q_scb_calc/1(EORthrustECI)  "vec_eci"
  Quaternion Inverse/1 -> Quaternion Rotation/1
  q_scb_calc/1(qECI2scbp) -> Quaternion Multiplication/1
  Flipsign/1 -> Subsystem/2(Flipsign)
  Subsystem/1(qscbp2scb) -> Quaternion Multiplication/2
  EORthrustSCB/1 -> Subsystem/1(EORthrustSCB)  "thrustscb"
  Quaternion Multiplication/1 -> qECI2scb/1

== system HSat_orbit/Subsystem1/Subsystem4/EORattitude/Subsystem/Subsystem3 ==
  AmomSCB : Inport
  EORtorqueSCB : Inport  Port=2
  FlipSatellite : Subsystem
  Subsystem : Subsystem
  DoAMOM : Outport
  NoAMOM : Outport  Port=2
  FlipPlusMinus : Outport  Port=3
  wires:
  AmomSCB/1 -> FlipSatellite/1(AmomSCB)
  Subsystem/1(FlipPlusMinus) -> FlipPlusMinus/1
  EORtorqueSCB/1 -> FlipSatellite/2(EORtorqueSCB)
  FlipSatellite/1(FlipSatellite_bool) -> Subsystem/1(FlipNow)
  FlipSatellite/2(DoAMOM) -> DoAMOM/1
  FlipSatellite/3(NoAMOM) -> NoAMOM/1

== system HSat_orbit/Subsystem1/Subsystem4/EORattitude/Subsystem2/PPU1 ==
  ForceORSCB : Inport
  OR ThrustNo : Inport  Port=2
  TorqueORSCB : Inport  Port=3
  Constant : Constant  Value=[0 0 0 0 0 0 0 0 1 0 0]
  Constant1 : Constant  Value=[0 0 0 0 0 0 0 0 0 0 0]
  Constant2 : Constant  Value=[0 0 0 0 0 0 0 0 0 0 1]
  Demux : Demux  Outputs=3
  Demux1 : Demux  Outputs=3
  Multiport Switch : MultiPortSwitch  SaturateOnIntegerOverflow=off  InputSameDT=off
  Multiport Switch1 : MultiPortSwitch  SaturateOnIntegerOverflow=off  InputSameDT=off
  Multiport Switch2 : MultiPortSwitch  SaturateOnIntegerOverflow=off  InputSameDT=off
  ForceSCB : Outport
  TorqueSCB : Outport  Port=2
  activethrusters : Outport  Port=3
  wires:
  ForceORSCB/1 -> Demux/1
  Demux/1 -> Multiport Switch/2
  Demux/2 -> Multiport Switch/3
  Demux/3 -> Multiport Switch/4
  Multiport Switch/1 -> ForceSCB/1
  Constant1/1 -> Multiport Switch1/3
  Multiport Switch1/1 -> activethrusters/1
  Constant/1 -> Multiport Switch1/2
  Constant2/1 -> Multiport Switch1/4
  Multiport Switch2/1 -> TorqueSCB/1
  TorqueORSCB/1 -> Demux1/1
  Demux1/3 -> Multiport Switch2/4
  Demux1/1 -> Multiport Switch2/2
  OR ThrustNo/1 -> Multiport Switch1/1, Multiport Switch2/1, Multiport Switch/1
  Demux1/2 -> Multiport Switch2/3

== system HSat_orbit/Subsystem1/Subsystem4/EORattitude/Subsystem2/PPU3 ==
  ForceORSCB : Inport
  OR ThrustNo : Inport  Port=2
  TorqueORSCB : Inport  Port=3
  Constant : Constant  Value=[0 0 0 0 0 0 0 0 0 0 0]
  Constant1 : Constant  Value=[0 0 0 0 0 0 0 0 0 1 0]
  Constant2 : Constant  Value=[0 0 0 0 0 0 0 0 0 0 1]
  Demux : Demux  Outputs=3
  Demux1 : Demux  Outputs=3
  Multiport Switch : MultiPortSwitch  SaturateOnIntegerOverflow=off  InputSameDT=off
  Multiport Switch1 : MultiPortSwitch  SaturateOnIntegerOverflow=off  InputSameDT=off
  Multiport Switch2 : MultiPortSwitch  SaturateOnIntegerOverflow=off  InputSameDT=off
  ForceSCB : Outport
  TorqueSCB : Outport  Port=2
  activethrusters : Outport  Port=3
  wires:
  ForceORSCB/1 -> Demux/1
  Demux/1 -> Multiport Switch/2
  Demux/2 -> Multiport Switch/3
  Demux/3 -> Multiport Switch/4
  Multiport Switch/1 -> ForceSCB/1
  Constant1/1 -> Multiport Switch1/3
  Multiport Switch1/1 -> activethrusters/1
  Constant/1 -> Multiport Switch1/2
  Constant2/1 -> Multiport Switch1/4
  Multiport Switch2/1 -> TorqueSCB/1
  TorqueORSCB/1 -> Demux1/1
  Demux1/3 -> Multiport Switch2/4
  Demux1/1 -> Multiport Switch2/2
  OR ThrustNo/1 -> Multiport Switch1/1, Multiport Switch2/1, Multiport Switch/1
  Demux1/2 -> Multiport Switch2/3

== system HSat_orbit/Subsystem1/Subsystem4/EORattitude/Subsystem2/Subsystem1 ==
  AllForcesSCB : Inport
  AllTorquesSCB : Inport  Port=2
  ForceSCBOR1 : Selector  NumberOfDimensions=2  InputPortWidth=3  IndexOptions=Index vector (dialog),Index vector (dialog)  Indices=9,[1 2 3]  OutputSizes=1,1
  ForceSCBOR2 : Selector  NumberOfDimensions=2  InputPortWidth=3  IndexOptions=Index vector (dialog),Index vector (dialog)  Indices=10,[1 2 3]  OutputSizes=1,1
  ForceSCBOR3 : Selector  NumberOfDimensions=2  InputPortWidth=3  IndexOptions=Index vector (dialog),Index vector (dialog)  Indices=11,[1 2 3]  OutputSizes=1,1
  Mux : Mux  Inputs=3
  Mux1 : Mux  Inputs=3
  TorqueSCBOR4 : Selector  NumberOfDimensions=2  InputPortWidth=3  IndexOptions=Index vector (dialog),Index vector (dialog)  Indices=9,[1 2 3]  OutputSizes=1,1
  TorqueSCBOR5 : Selector  NumberOfDimensions=2  InputPortWidth=3  IndexOptions=Index vector (dialog),Index vector (dialog)  Indices=10,[1 2 3]  OutputSizes=1,1
  TorqueSCBOR6 : Selector  NumberOfDimensions=2  InputPortWidth=3  IndexOptions=Index vector (dialog),Index vector (dialog)  Indices=11,[1 2 3]  OutputSizes=1,1
  ForceORSCB : Outport
  TorquesORSCB : Outport  Port=2
  wires:
  ForceSCBOR3/1 -> Mux/3
  ForceSCBOR2/1 -> Mux/2
  ForceSCBOR1/1 -> Mux/1
  AllForcesSCB/1 -> ForceSCBOR2/1, ForceSCBOR3/1, ForceSCBOR1/1
  Mux/1 -> ForceORSCB/1
  Mux1/1 -> TorquesORSCB/1
  TorqueSCBOR4/1 -> Mux1/1
  TorqueSCBOR5/1 -> Mux1/2
  AllTorquesSCB/1 -> TorqueSCBOR5/1, TorqueSCBOR6/1, TorqueSCBOR4/1
  TorqueSCBOR6/1 -> Mux1/3

== system HSat_orbit/Subsystem1/Subsystem4/EORattitude/Subsystem4/Subsystem1 ==
  q : Inport
  vec : Inport  Port=2
  sunvECI : Inport  Port=3
  thrustscb : Inport  Port=4
  Quaternion Inverse : aerolibutil/Quaternion Inverse
  Quaternion Multiplication : aerolibutil/Quaternion Multiplication
  Quaternion Rotation : aerolibutil/Quaternion Rotation
  Subsystem : Subsystem
  q_scb_calc : Subsystem
  q*r : Outport
  wires:
  q/1 -> Quaternion Inverse/1
  Quaternion Multiplication/1 -> q*r/1
  sunvECI/1 -> q_scb_calc/2(sunvECI)
  q_scb_calc/1(qECI2scbp) -> Quaternion Multiplication/1
  thrustscb/1 -> Subsystem/1(EORthrustSCB)
  Quaternion Inverse/1 -> Quaternion Rotation/1
  Subsystem/1(qscbp2scb) -> Quaternion Multiplication/2
  vec/1 -> Quaternion Rotation/2
  Quaternion Rotation/1 -> q_scb_calc/1(EORthrustECI)  "vec_eci"

== system HSat_orbit/Subsystem1/Subsystem4/EORattitude/Subsystem4/Subsystem2 ==
  thrustscb : Inport
  Constant : Constant  Value=0
  VecNormalize4 : Subsystem
      mask Display: disp('u/||u||')
  Vector Concatenate : Concatenate
  qflipscb : Outport
  wires:
  thrustscb/1 -> VecNormalize4/1(In1)
  Vector Concatenate/1 -> qflipscb/1
  Constant/1 -> Vector Concatenate/1
  VecNormalize4/1(Out1) -> Vector Concatenate/2  "zscbpSCB"

== system HSat_orbit/Subsystem1/Subsystem4/EORattitude/Subsystem4/Subsystem3 ==
  AmomSCB : Inport
  EORtorqueSCB : Inport  Port=2
  FlipSatellite : Subsystem
  Subsystem : Subsystem
  Flipyaxis : Outport
  DoAMOM : Outport  Port=2
  NoAMOM : Outport  Port=3
  wires:
  AmomSCB/1 -> FlipSatellite/1(AmomSCB)
  Subsystem/1(FlipPlusMinus) -> Flipyaxis/1
  EORtorqueSCB/1 -> FlipSatellite/2(EORtorqueSCB)
  FlipSatellite/1(FlipSatellite_bool) -> Subsystem/1(FlipNow)
  FlipSatellite/2(DoAMOM) -> DoAMOM/1
  FlipSatellite/3(NoAMOM) -> NoAMOM/1

== system HSat_orbit/Subsystem1/Subsystem4/EORattitude/Subsystem4/Subsystem4 ==
  Constant : Constant  Value=[1 0 0 0]
  qflipscb : Outport
  wires:
  Constant/1 -> qflipscb/1

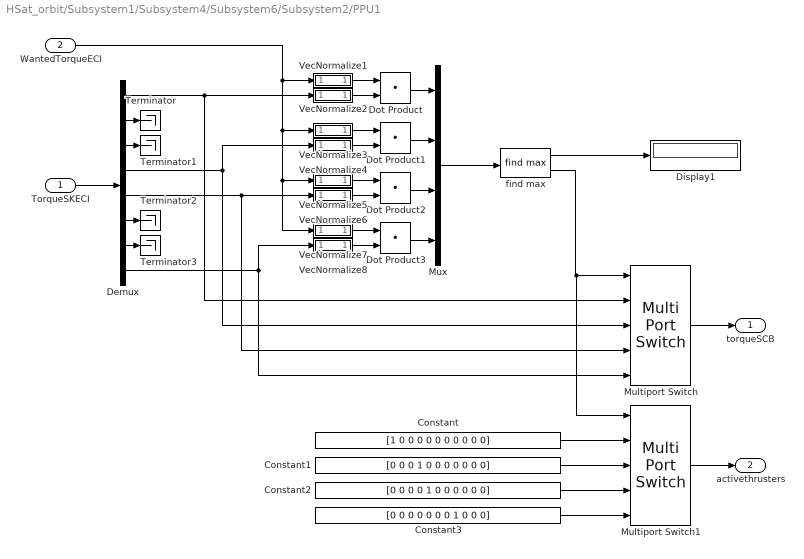
== system HSat_orbit/Subsystem1/Subsystem4/Subsystem6/Subsystem2/PPU1 ==
  TorqueSKECI : Inport
  WantedTorqueECI : Inport  Port=2
  Constant : Constant  Value=[1 0 0 0 0 0 0 0 0 0 0]
  Constant1 : Constant  Value=[0 0 0 1 0 0 0 0 0 0 0]
  Constant2 : Constant  Value=[0 0 0 0 1 0 0 0 0 0 0]
  Constant3 : Constant  Value=[0 0 0 0 0 0 0 1 0 0 0]
  Demux : Demux  Outputs=8
  Display1 : Display
  Dot Product{,1..3} (4 alike) : DotProduct  OutDataTypeStr=Inherit: Inherit via internal rule
  Multiport Switch : MultiPortSwitch  Inputs=4  SaturateOnIntegerOverflow=off  InputSameDT=off
  Multiport Switch1 : MultiPortSwitch  Inputs=4  SaturateOnIntegerOverflow=off  InputSameDT=off
  Mux : Mux
  Terminator{,1..3} (4 alike) : Terminator
  VecNormalize1 : Subsystem
      mask Display: disp('u/||u||')
  VecNormalize2 : Subsystem
      mask Display: disp('u/||u||')
  VecNormalize3 : Subsystem
      mask Display: disp('u/||u||')
  VecNormalize4 : Subsystem
      mask Display: disp('u/||u||')
  VecNormalize5 : Subsystem
      mask Display: disp('u/||u||')
  VecNormalize6 : Subsystem
      mask Display: disp('u/||u||')
  VecNormalize7 : Subsystem
      mask Display: disp('u/||u||')
  VecNormalize8 : Subsystem
      mask Display: disp('u/||u||')
  find max : Toolbox/vector blocks/find max  SystemSampleTime=-1  VariantActivationTime=update diagram  Latency=0  AutoFrameSizeCalculation=off
      settings: SourceProductName=SSC flight toolbox
  torqueSCB : Outport
  activethrusters : Outport  Port=2
  wires:
  TorqueSKECI/1 -> Demux/1
  Demux/2 -> Terminator/1
  Demux/3 -> Terminator1/1
  Demux/6 -> Terminator2/1
  Demux/7 -> Terminator3/1
  Demux/1 -> Multiport Switch/2, VecNormalize2/1(In1)
  Demux/4 -> Multiport Switch/3, VecNormalize4/1(In1)
  Demux/5 -> Multiport Switch/4, VecNormalize6/1(In1)
  Demux/8 -> Multiport Switch/5, VecNormalize8/1(In1)
  WantedTorqueECI/1 -> VecNormalize1/1(In1), VecNormalize3/1(In1), VecNormalize5/1(In1), VecNormalize7/1(In1)
  VecNormalize1/1(Out1) -> Dot Product/1
  VecNormalize2/1(Out1) -> Dot Product/2
  VecNormalize3/1(Out1) -> Dot Product1/1
  VecNormalize4/1(Out1) -> Dot Product1/2
  VecNormalize5/1(Out1) -> Dot Product2/1
  VecNormalize6/1(Out1) -> Dot Product2/2
  VecNormalize7/1(Out1) -> Dot Product3/1
  VecNormalize8/1(Out1) -> Dot Product3/2
  Dot Product/1 -> Mux/1
  Dot Product1/1 -> Mux/2
  Dot Product2/1 -> Mux/3
  Dot Product3/1 -> Mux/4
  Mux/1 -> find max/1
  find max/2 -> Multiport Switch1/1, Multiport Switch/1
  find max/1 -> Display1/1
  Multiport Switch/1 -> torqueSCB/1
  Constant/1 -> Multiport Switch1/2
  Constant1/1 -> Multiport Switch1/3
  Constant2/1 -> Multiport Switch1/4
  Constant3/1 -> Multiport Switch1/5
  Multiport Switch1/1 -> activethrusters/1

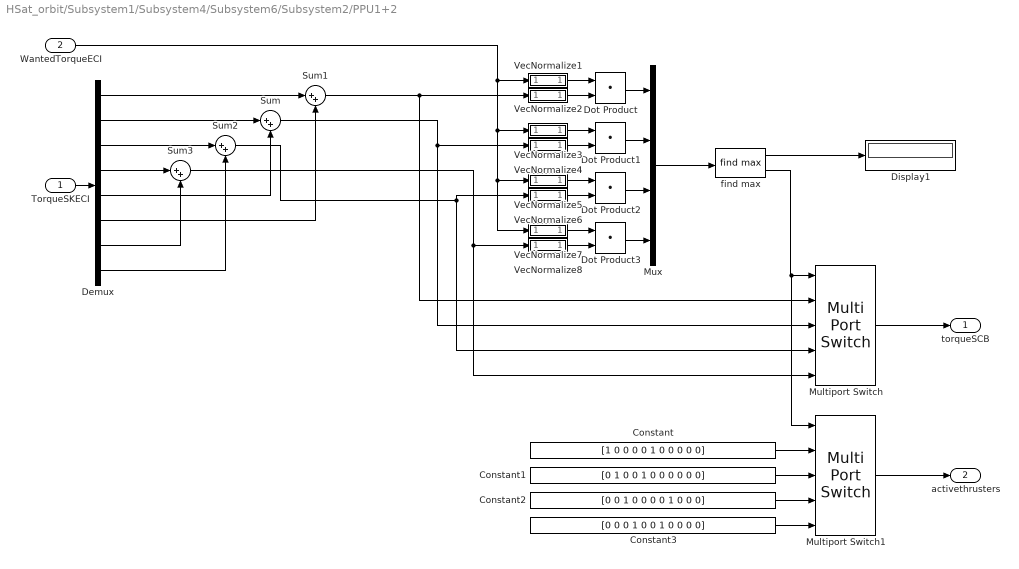
== system HSat_orbit/Subsystem1/Subsystem4/Subsystem6/Subsystem2/PPU1+2 ==
  TorqueSKECI : Inport
  WantedTorqueECI : Inport  Port=2
  Constant : Constant  Value=[1 0 0 0 0 1 0 0 0 0 0]
  Constant1 : Constant  Value=[0 1 0 0 1 0 0 0 0 0 0]
  Constant2 : Constant  Value=[0 0 1 0 0 0 0 1 0 0 0]
  Constant3 : Constant  Value=[0 0 0 1 0 0 1 0 0 0 0]
  Demux : Demux  Outputs=8
  Display1 : Display
  Dot Product{,1..3} (4 alike) : DotProduct  OutDataTypeStr=Inherit: Inherit via internal rule
  Multiport Switch : MultiPortSwitch  Inputs=4  SaturateOnIntegerOverflow=off  InputSameDT=off
  Multiport Switch1 : MultiPortSwitch  Inputs=4  SaturateOnIntegerOverflow=off  InputSameDT=off
  Mux : Mux
  Sum{,1..3} (4 alike) : Sum  Inputs=|++
  VecNormalize1 : Subsystem
      mask Display: disp('u/||u||')
  VecNormalize2 : Subsystem
      mask Display: disp('u/||u||')
  VecNormalize3 : Subsystem
      mask Display: disp('u/||u||')
  VecNormalize4 : Subsystem
      mask Display: disp('u/||u||')
  VecNormalize5 : Subsystem
      mask Display: disp('u/||u||')
  VecNormalize6 : Subsystem
      mask Display: disp('u/||u||')
  VecNormalize7 : Subsystem
      mask Display: disp('u/||u||')
  VecNormalize8 : Subsystem
      mask Display: disp('u/||u||')
  find max : Toolbox/vector blocks/find max  SystemSampleTime=-1  VariantActivationTime=update diagram  Latency=0  AutoFrameSizeCalculation=off
      settings: SourceProductName=SSC flight toolbox
  torqueSCB : Outport
  activethrusters : Outport  Port=2
  wires:
  TorqueSKECI/1 -> Demux/1
  Sum1/1 -> Multiport Switch/2, VecNormalize2/1(In1)
  Sum/1 -> Multiport Switch/3, VecNormalize4/1(In1)
  Sum2/1 -> Multiport Switch/4, VecNormalize6/1(In1)
  Sum3/1 -> Multiport Switch/5, VecNormalize8/1(In1)
  WantedTorqueECI/1 -> VecNormalize1/1(In1), VecNormalize3/1(In1), VecNormalize5/1(In1), VecNormalize7/1(In1)
  VecNormalize1/1(Out1) -> Dot Product/1
  VecNormalize2/1(Out1) -> Dot Product/2
  VecNormalize3/1(Out1) -> Dot Product1/1
  VecNormalize4/1(Out1) -> Dot Product1/2
  VecNormalize5/1(Out1) -> Dot Product2/1
  VecNormalize6/1(Out1) -> Dot Product2/2
  VecNormalize7/1(Out1) -> Dot Product3/1
  VecNormalize8/1(Out1) -> Dot Product3/2
  Dot Product/1 -> Mux/1
  Dot Product1/1 -> Mux/2
  Dot Product2/1 -> Mux/3
  Dot Product3/1 -> Mux/4
  Mux/1 -> find max/1
  find max/1 -> Display1/1
  Multiport Switch/1 -> torqueSCB/1
  Demux/4 -> Sum3/1
  Demux/1 -> Sum1/1
  Demux/2 -> Sum/1
  Demux/3 -> Sum2/1
  Demux/6 -> Sum1/2
  Demux/5 -> Sum/2
  Demux/8 -> Sum2/2
  Demux/7 -> Sum3/2
  Constant3/1 -> Multiport Switch1/5
  find max/2 -> Multiport Switch1/1, Multiport Switch/1
  Constant1/1 -> Multiport Switch1/3
  Multiport Switch1/1 -> activethrusters/1
  Constant/1 -> Multiport Switch1/2
  Constant2/1 -> Multiport Switch1/4
